simulink model "Single1"  (Simulink 6.0)
settings: Solver=ode45  StartTime=0.0  StopTime=10.0  RelTol=1e-3
settings Model: Creator=scaife  LastModifiedBy=scaife  ExtModeAutoUpdateStatusClock=off

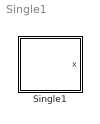
== system Single1 ==
  Single1 : Stateflow chart

== stateflow chart Single1 ==
  state A/
    du: x++;
  data: x output double
